simulink model "Openloop_voltage_control"  (R2020b)
settings: Solver=FixedStepDiscrete  StartTime=0.0  StopTime=Inf  RelTol=1e-3  EnableMultiTasking=on
values from neighbouring files (symbols this model uses):
  D_IGBT_CCM = (V_IGBT_out+V_diode_forward_drop-V_in)/(V_IGBT_out+V_diode_forward_drop)    (= 0.850746268657)    [Openloop_voltage_control_parameters.m]
  D_MOSFET_CCM = (V_MOSFET_out+V_diode_forward_drop-V_in)/(V_MOSFET_out+V_diode_forward_drop)    (= 0.70297029703)    [Openloop_voltage_control_parameters.m]
  Ki_IGBT = 0    [Openloop_voltage_control_parameters.m]
  Ki_MOSFET = 0    [Openloop_voltage_control_parameters.m]
  Kp_IGBT = 0    [Openloop_voltage_control_parameters.m]
  Kp_MOSFET = 0    [Openloop_voltage_control_parameters.m]
  Timer_period_IGBT = round(60e6/f_sw_IGBT)    [Openloop_voltage_control_parameters.m]
  Timer_period_MOSFET = round(60e6/f_sw_MOSFET)    [Openloop_voltage_control_parameters.m]
undefined symbols (not defined in the file or in its folder): GPTRIP1SEL, GPTRIP2SEL, TZ1, TZ2
undefined symbols (not defined in the file): C2000, Clear, Disable, ePWM2, ePWMxA, Immediate, Positive, Set, Up
libraries: c2802xlib x9, pid_lib x2, dspsigops x2, c280xlib x1
(part 1 of 2)
settings Model: ExtModeTrigDuration=8  Creator=Mladen  LastModifiedBy=hites
settings SolverCC: AutoInsertRateTranBlk=on
settings DataIOCC: ReturnWorkspaceOutputs=off
settings OptimizationCC: DefaultUnderspecifiedDataType=single  EnhancedBackFolding=on  PassReuseOutputArgsAs=Individual arguments  MaxStackSize=512  OptimizeBlockOrder=speed  DifferentSizesBufferReuse=on  OptimizationCustomize=off  EfficientTunableParamExpr=on
settings DebuggingCC: ParameterTunabilityLossMsg=error  ArithmeticOperatorsInVariantConditions=warning
settings HardwareCC: ProdBitPerChar=16  ProdBitPerInt=16  ProdBitPerPointer=32  ProdBitPerSizeT=32  ProdBitPerPtrDiffT=32  ProdLargestAtomicInteger=Integer  ProdLargestAtomicFloat=None  ProdWordSize=16  ProdLongLongMode=on  ProdHWDeviceType=Texas Instruments->C2000
settings SFSimCC: MATLABDynamicMemAlloc=off  CustomCodeUndefinedFunction=UseInterfaceOnly
settings RTWCC: Description=Embedded Coder  SystemTargetFile=ert.tlc  HardwareBoard=TI Piccolo F28027/F28027F LaunchPad  TemplateMakefile=ert_default_tmf  GenerateReport=on  Toolchain=Texas Instruments Code Composer Studio (C2000)  IncludeHyperlinkInReport=on  LaunchReport=on  GenerateTraceInfo=on  GenerateTraceReport=on  GenerateTraceReportSl=on  GenerateTraceReportSf=on  GenerateTraceReportEml=on
settings CodeAppCC: ForceParamTrailComments=on  IgnoreCustomStorageClasses=off  OperatorAnnotations=on  SimulinkDataObjDesc=on  SFDataObjDesc=on  InsertBlockDesc=on
settings ERTTargetCC: CodeReplacementLibrary=TI C28x

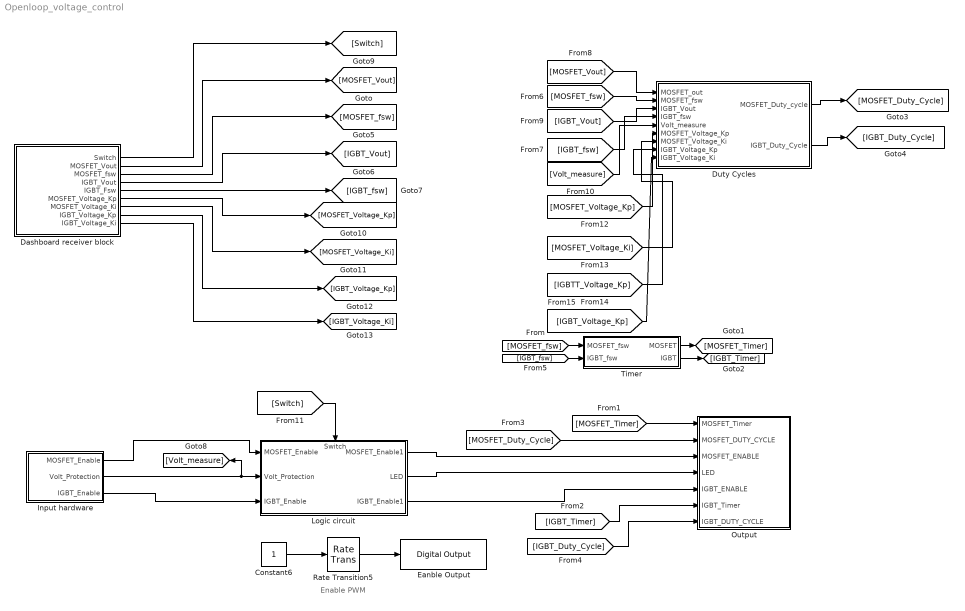
== system Openloop_voltage_control ==
  note: Enable PWM
  Constant6 : Constant  OutDataTypeStr=boolean  SampleTime=0.01
  Dashboard receiver block : Subsystem
  Duty Cycles : Subsystem
  Eanble Output : c2802xlib/Digital Output  GPIO_Number=GPIO0~GPIO7  GPIO_Bit0=off  GPIO_BIT0_Toggle=off  GPIO_Bit1=off  GPIO_BIT1_Toggle=off  GPIO_Bit2=off  GPIO_BIT2_Toggle=off  GPIO_Bit3=off  GPIO_BIT3_Toggle=off  GPIO_Bit4=on  GPIO_BIT4_Toggle=off  GPIO_Bit5=off  GPIO_BIT5_Toggle=off  GPIO_Bit6=off  GPIO_BIT6_Toggle=off  GPIO_Bit7=off  GPIO_BIT7_Toggle=off
      settings: SourceProductBaseCode=TIC2000
  Input hardware : Subsystem
  Logic circuit : Subsystem
      settings: PortSchema="{\"entries\":[{\"content\":{\"sides\":[{\"content\":{\"connectorIds\":[\"In1\",\"In2\",\"In3\"]},\"type\":\"ConnectorPlacement.EquallySpacedRectSide\",\"uuid\":\"9edef9f6-4e06-49ff-9487-f0c876c6db56\"},{\"content\":{\"connectorIds\":[\"Out1\",\"Out2\",\"Out3\"],\"side\":\"RIGHT\"},\"type\":\"ConnectorPlacement.EquallySpacedRectSide\",\"uuid\":\"38654259-1306-4cb6-b452-8646906e5123\"},{\"content\":{\"connectorIds\":[\"In4\"],\"side\":\"TOP\"},\"type\":\"ConnectorPlacement.EquallySpacedRectSide\",\"uuid\":\"81b5187c-2f62-4987-b311-955428575483\"},{\"content\":{\"connectorIds\":[],\"side\":\"HIDDEN\"},\"type\":\"ConnectorPlacement.EquallySpacedRectSide\",\"uuid\":\"52992d09-5af1-4048-a992-404c39f4bc87\"}]},\"type\":\"ConnectorPlacement.EquallySpacedConnector\",\"uuid\":\"3860a4b4-3099-482c-9336-e0768bc23cc0\"}],\"packageUris\":[\"http://schema.mathworks.com/mf0/Connector/R2020b\"],\"version\":\"1.0\"}"
  Output : Subsystem
  Rate Transition5 : RateTransition  Deterministic=off
  Timer : Subsystem
  wires:
  Constant6/1 -> Rate Transition5/1
  Rate Transition5/1 -> Eanble Output/1
  Duty Cycles/1(MOSFET_Duty_cycle) -> [MOSFET_Duty_Cycle]
  Duty Cycles/2(IGBT_Duty_Cycle) -> [IGBT_Duty_Cycle]
  Timer/1(MOSFET) -> [MOSFET_Timer]
  Timer/2(IGBT) -> [IGBT_Timer]
  Dashboard receiver block/2(MOSFET_Vout) -> [MOSFET_Vout]
  Dashboard receiver block/3(MOSFET_fsw) -> [MOSFET_fsw]
  Dashboard receiver block/4(IGBT_Vout) -> [IGBT_Vout]
  Dashboard receiver block/5(IGBT_Fsw) -> [IGBT_fsw]
  [MOSFET_fsw] -> Timer/1(MOSFET_fsw)
  [IGBT_fsw] -> Timer/2(IGBT_fsw)
  [MOSFET_Vout] -> Duty Cycles/1(MOSFET_out)
  [MOSFET_fsw] -> Duty Cycles/2(MOSFET_fsw)
  [IGBT_Vout] -> Duty Cycles/3(IGBT_Vout)
  [IGBT_fsw] -> Duty Cycles/4(IGBT_fsw)
  [Volt_measure] -> Duty Cycles/5(Volt_measure)
  Input hardware/2(Volt_Protection) -> [Volt_measure], Logic circuit/2(Volt_Protection)
  Input hardware/1(MOSFET_Enable) -> Logic circuit/1(MOSFET_Enable)
  Input hardware/3(IGBT_Enable) -> Logic circuit/3(IGBT_Enable)
  [MOSFET_Timer] -> Output/1(MOSFET_Timer)
  [MOSFET_Duty_Cycle] -> Output/2(MOSFET_DUTY_CYCLE)
  Logic circuit/1(MOSFET_Enable1) -> Output/3(MOSFET_ENABLE)
  Logic circuit/2(LED) -> Output/4(LED)
  Logic circuit/3(IGBT_Enable1) -> Output/5(IGBT_ENABLE)
  [IGBT_Timer] -> Output/6(IGBT_Timer)
  [IGBT_Duty_Cycle] -> Output/7(IGBT_DUTY_CYCLE)
  Dashboard receiver block/1(Switch) -> [Switch]
  Dashboard receiver block/6(MOSFET_Voltage_Kp) -> [MOSFET_Voltage_Kp]
  Dashboard receiver block/7(MOSFET_Voltage_Ki) -> [MOSFET_Voltage_Ki]
  Dashboard receiver block/8(IGBT_Voltage_Kp) -> [IGBT_Voltage_Kp]
  Dashboard receiver block/9(IGBT_Voltage_Ki) -> [IGBT_Voltage_Ki]
  [Switch] -> Logic circuit/4(Switch)
  [MOSFET_Voltage_Ki] -> Duty Cycles/7(MOSFET_Voltage_Ki)
  [MOSFET_Voltage_Kp] -> Duty Cycles/6(MOSFET_Voltage_Kp)
  [IGBTT_Voltage_Kp] -> Duty Cycles/8(IGBT_Voltage_Kp)
  [IGBT_Voltage_Kp] -> Duty Cycles/9(IGBT_Voltage_Ki)

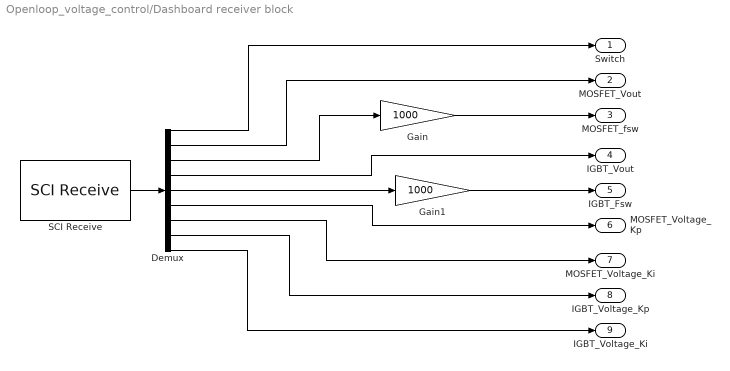
== system Openloop_voltage_control/Dashboard receiver block ==
  Demux : Demux  Outputs=9
  Gain : Gain  Gain=1000
  Gain1 : Gain  Gain=1000
  SCI Receive : c280xlib/SCI Receive  sciModule=A  dataHead='S'  dataTail='E'  dataType=uint16  dataDim=9  initValue=0  errOption=Output the last received value  errValue=0  sampleTime=-1  outputStatus=off  postInterrupt=off  numFifo=1
      settings: SourceProductName=Embedded Coder Support Package for Texas Instruments C2000 Processors
  Switch : Outport
  MOSFET_Vout : Outport  Port=2
  MOSFET_fsw : Outport  Port=3
  IGBT_Vout : Outport  Port=4
  IGBT_Fsw : Outport  Port=5
  MOSFET_Voltage_Kp : Outport  Port=6
  MOSFET_Voltage_Ki : Outport  Port=7
  IGBT_Voltage_Kp : Outport  Port=8
  IGBT_Voltage_Ki : Outport  Port=9
  wires:
  SCI Receive/1 -> Demux/1
  Gain/1 -> MOSFET_fsw/1
  Gain1/1 -> IGBT_Fsw/1
  Demux/5 -> Gain1/1
  Demux/4 -> IGBT_Vout/1
  Demux/3 -> Gain/1
  Demux/2 -> MOSFET_Vout/1
  Demux/1 -> Switch/1
  Demux/7 -> MOSFET_Voltage_Ki/1
  Demux/8 -> IGBT_Voltage_Kp/1
  Demux/9 -> IGBT_Voltage_Ki/1
  Demux/6 -> MOSFET_Voltage_Kp/1

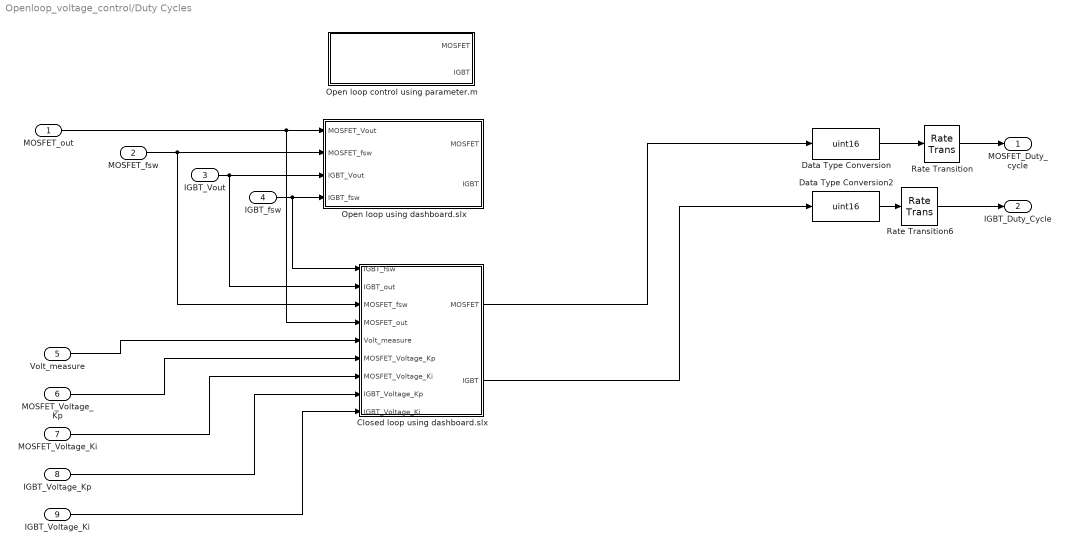
== system Openloop_voltage_control/Duty Cycles ==
  MOSFET_out : Inport
  MOSFET_fsw : Inport  Port=2
  IGBT_Vout : Inport  Port=3
  IGBT_fsw : Inport  Port=4
  Volt_measure : Inport  Port=5
  MOSFET_Voltage_Kp : Inport  Port=6
  MOSFET_Voltage_Ki : Inport  Port=7
  IGBT_Voltage_Kp : Inport  Port=8
  IGBT_Voltage_Ki : Inport  Port=9
  Closed loop using dashboard.slx : Subsystem
  Data Type Conversion : DataTypeConversion  OutDataTypeStr=uint16
  Data Type Conversion2 : DataTypeConversion  OutDataTypeStr=uint16
  Open loop control using parameter.m : Subsystem
  Open loop using dashboard.slx : Subsystem
  Rate Transition : RateTransition
  Rate Transition6 : RateTransition
  MOSFET_Duty_cycle : Outport
  IGBT_Duty_Cycle : Outport  Port=2
  wires:
  Data Type Conversion/1 -> Rate Transition/1
  Rate Transition/1 -> MOSFET_Duty_cycle/1
  Data Type Conversion2/1 -> Rate Transition6/1
  Rate Transition6/1 -> IGBT_Duty_Cycle/1
  MOSFET_out/1 -> Closed loop using dashboard.slx/4(MOSFET_out), Open loop using dashboard.slx/1(MOSFET_Vout)
  MOSFET_fsw/1 -> Closed loop using dashboard.slx/3(MOSFET_fsw), Open loop using dashboard.slx/2(MOSFET_fsw)
  IGBT_Vout/1 -> Closed loop using dashboard.slx/2(IGBT_out), Open loop using dashboard.slx/3(IGBT_Vout)
  IGBT_fsw/1 -> Closed loop using dashboard.slx/1(IGBT_fsw), Open loop using dashboard.slx/4(IGBT_fsw)
  Volt_measure/1 -> Closed loop using dashboard.slx/5(Volt_measure)
  MOSFET_Voltage_Kp/1 -> Closed loop using dashboard.slx/6(MOSFET_Voltage_Kp)
  MOSFET_Voltage_Ki/1 -> Closed loop using dashboard.slx/7(MOSFET_Voltage_Ki)
  IGBT_Voltage_Kp/1 -> Closed loop using dashboard.slx/8(IGBT_Voltage_Kp)
  IGBT_Voltage_Ki/1 -> Closed loop using dashboard.slx/9(IGBT_Voltage_Ki)
  Closed loop using dashboard.slx/1(MOSFET) -> Data Type Conversion/1
  Closed loop using dashboard.slx/2(IGBT) -> Data Type Conversion2/1

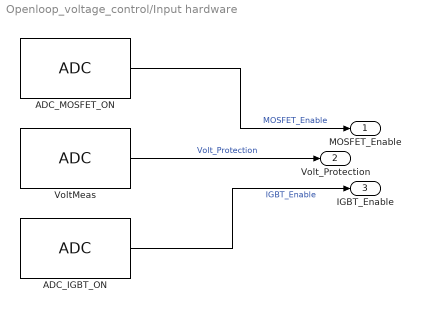
== system Openloop_voltage_control/Input hardware ==
  ADC_IGBT_ON : c2802xlib/ADC  blkParamProc=C2000  ADCModule=1  samplingMode=Single sample mode  ADCResolution=12-bit (Single-ended input)  useSOC1=SOC2  useSOC2=SOC0_SOC1  SOCAcquisitionWindow=7  SOCTriggerSource=Software  SOCInterruptTrigger=No ADCINT  Ts=0.001  dType=uint16  postInterrupt=off  interruptSel=ADCINT1  ADCINTContinuous=off  endma=off  chdma=1  conv1=ADCINA3  conv2=ADCINA7 and ADCINB7  conv1_Type4=ADCIN0  conv2_Type4=ADCIN0 and ADCIN1
  ADC_MOSFET_ON : c2802xlib/ADC  blkParamProc=C2000  ADCModule=1  samplingMode=Single sample mode  ADCResolution=12-bit (Single-ended input)  useSOC1=SOC0  useSOC2=SOC0_SOC1  SOCAcquisitionWindow=7  SOCTriggerSource=Software  SOCInterruptTrigger=No ADCINT  Ts=0.001  dType=uint16  postInterrupt=off  interruptSel=ADCINT1  ADCINTContinuous=off  endma=off  chdma=1  conv1=ADCINA7  conv2=ADCINA7 and ADCINB7  conv1_Type4=ADCIN0  conv2_Type4=ADCIN0 and ADCIN1
  VoltMeas : c2802xlib/ADC  blkParamProc=C2000  ADCModule=1  samplingMode=Single sample mode  ADCResolution=12-bit (Single-ended input)  useSOC1=SOC8  useSOC2=SOC0_SOC1  SOCAcquisitionWindow=7  SOCTriggerSource=Software  SOCInterruptTrigger=No ADCINT  Ts=0.001  dType=uint16  postInterrupt=off  interruptSel=ADCINT1  ADCINTContinuous=off  endma=off  chdma=1  conv1=ADCINB1  conv2=ADCINA7 and ADCINB7  conv1_Type4=ADCIN0  conv2_Type4=ADCIN0 and ADCIN1
  MOSFET_Enable : Outport
  Volt_Protection : Outport  Port=2
  IGBT_Enable : Outport  Port=3
  wires:
  ADC_MOSFET_ON/1 -> MOSFET_Enable/1  "MOSFET_Enable"
  VoltMeas/1 -> Volt_Protection/1  "Volt_Protection"
  ADC_IGBT_ON/1 -> IGBT_Enable/1  "IGBT_Enable"

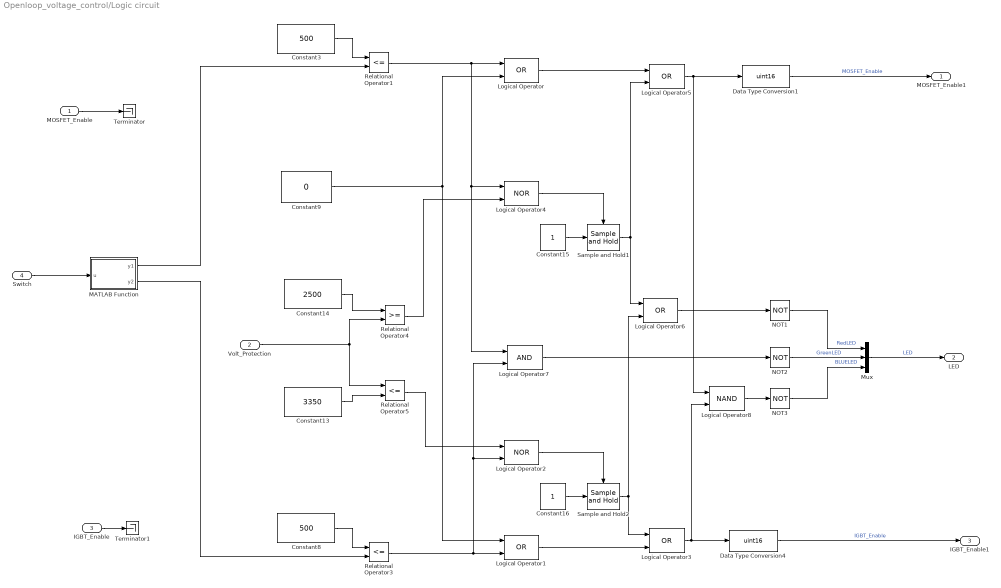
== system Openloop_voltage_control/Logic circuit ==
  MOSFET_Enable : Inport
  Volt_Protection : Inport  Port=2
  IGBT_Enable : Inport  Port=3
  Switch : Inport  Port=4
  Constant13 : Constant  Value=3350  OutDataTypeStr=uint16  SampleTime=-1
  Constant14 : Constant  Value=2500  OutDataTypeStr=uint16  SampleTime=-1
  Constant15 : Constant  OutDataTypeStr=boolean  SampleTime=-1
  Constant16 : Constant  OutDataTypeStr=boolean  SampleTime=-1
  Constant3 : Constant  Value=500  OutDataTypeStr=uint16  SampleTime=-1
  Constant8 : Constant  Value=500  OutDataTypeStr=uint16  SampleTime=-1
  Constant9 : Constant  Value=0  OutDataTypeStr=boolean  SampleTime=-1
  Data Type Conversion1 : DataTypeConversion  OutDataTypeStr=uint16
  Data Type Conversion4 : DataTypeConversion  OutDataTypeStr=uint16
  Logical Operator{,1,3,5..6} (5 alike) : Logic  Operator=OR  IconShape=distinctive  AllPortsSameDT=off  OutDataTypeStr=boolean
  Logical Operator2 : Logic  Operator=NOR  IconShape=distinctive  AllPortsSameDT=off  OutDataTypeStr=boolean
  Logical Operator4 : Logic  Operator=NOR  IconShape=distinctive  AllPortsSameDT=off  OutDataTypeStr=boolean
  Logical Operator7 : Logic  IconShape=distinctive  AllPortsSameDT=off  OutDataTypeStr=boolean
  Logical Operator8 : Logic  Operator=NAND  IconShape=distinctive  AllPortsSameDT=off  OutDataTypeStr=boolean
  MATLAB Function : MATLAB Function  TreatAsAtomicUnit=on
  Mux : Mux  Inputs=3
  NOT1 : Logic  Operator=NOT  IconShape=distinctive  AllPortsSameDT=off  OutDataTypeStr=boolean
  NOT2 : Logic  Operator=NOT  IconShape=distinctive  AllPortsSameDT=off  OutDataTypeStr=boolean
  NOT3 : Logic  Operator=NOT  IconShape=distinctive  AllPortsSameDT=off  OutDataTypeStr=boolean
  Relational Operator1 : RelationalOperator  Operator=<=  OutDataTypeStr=boolean  RndMeth=Simplest
  Relational Operator3 : RelationalOperator  Operator=<=  OutDataTypeStr=boolean  RndMeth=Simplest
  Relational Operator4 : RelationalOperator  OutDataTypeStr=boolean  RndMeth=Simplest
  Relational Operator5 : RelationalOperator  Operator=<=  OutDataTypeStr=boolean  RndMeth=Simplest
  Sample and Hold1 : dspsigops/Sample and Hold  trig=Rising edge  initCond=0  latchinput=off
  Sample and Hold2 : dspsigops/Sample and Hold  trig=Rising edge  initCond=0  latchinput=off
  Terminator : Terminator
  Terminator1 : Terminator
  MOSFET_Enable1 : Outport
  LED : Outport  Port=2
  IGBT_Enable1 : Outport  Port=3
  wires:
  Relational Operator1/1 -> Logical Operator7/1, Logical Operator4/1, Logical Operator/1
  Volt_Protection/1 -> Relational Operator4/2, Relational Operator5/1
  Logical Operator3/1 -> Data Type Conversion4/1, Logical Operator8/2
  Constant14/1 -> Relational Operator4/1
  Constant9/1 -> Logical Operator1/1, Logical Operator/2
  Logical Operator2/1 -> Sample and Hold2/Trigger
  Sample and Hold1/1 -> Logical Operator6/1, Logical Operator5/2
  Logical Operator5/1 -> Logical Operator8/1, Data Type Conversion1/1
  Constant15/1 -> Sample and Hold1/1
  Constant8/1 -> Relational Operator3/1
  Logical Operator8/1 -> NOT3/1
  Relational Operator3/1 -> Logical Operator7/2, Logical Operator2/2, Logical Operator1/2
  Data Type Conversion4/1 -> IGBT_Enable1/1  "IGBT_Enable"
  Logical Operator1/1 -> Logical Operator3/2
  Relational Operator4/1 -> Logical Operator4/2
  Logical Operator/1 -> Logical Operator5/1
  Relational Operator5/1 -> Logical Operator2/1
  Logical Operator4/1 -> Sample and Hold1/Trigger
  Sample and Hold2/1 -> Logical Operator3/1, Logical Operator6/2
  Constant3/1 -> Relational Operator1/1
  Constant16/1 -> Sample and Hold2/1
  Logical Operator7/1 -> NOT2/1
  Logical Operator6/1 -> NOT1/1
  Data Type Conversion1/1 -> MOSFET_Enable1/1  "MOSFET_Enable"
  NOT1/1 -> Mux/1  "RedLED"
  NOT2/1 -> Mux/2  "GreenLED"
  NOT3/1 -> Mux/3  "BLUELED"
  Mux/1 -> LED/1  "LED"
  Constant13/1 -> Relational Operator5/2
  Switch/1 -> MATLAB Function/1(u)
  MOSFET_Enable/1 -> Terminator/1
  IGBT_Enable/1 -> Terminator1/1
  MATLAB Function/1(y1) -> Relational Operator1/2
  MATLAB Function/2(y2) -> Relational Operator3/2

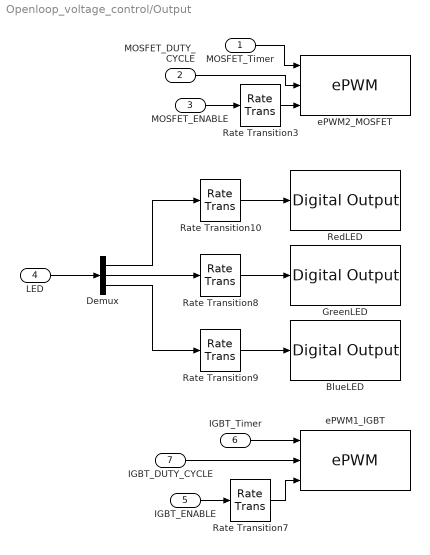
== system Openloop_voltage_control/Output ==
  MOSFET_Timer : Inport
  MOSFET_DUTY_CYCLE : Inport  Port=2
  MOSFET_ENABLE : Inport  Port=3
  LED : Inport  Port=4
  IGBT_ENABLE : Inport  Port=5
  IGBT_Timer : Inport  Port=6
  IGBT_DUTY_CYCLE : Inport  Port=7
  BlueLED : c2802xlib/Digital Output  GPIO_Number=GPIO8~GPIO15  GPIO_Bit0=off  GPIO_BIT0_Toggle=off  GPIO_Bit1=off  GPIO_BIT1_Toggle=off  GPIO_Bit2=off  GPIO_BIT2_Toggle=off  GPIO_Bit3=off  GPIO_BIT3_Toggle=off  GPIO_Bit4=on  GPIO_BIT4_Toggle=off  GPIO_Bit5=off  GPIO_BIT5_Toggle=off  GPIO_Bit6=off  GPIO_BIT6_Toggle=off  GPIO_Bit7=off  GPIO_BIT7_Toggle=off
      settings: SourceProductBaseCode=TIC2000
  Demux : Demux  Outputs=3
  GreenLED : c2802xlib/Digital Output  GPIO_Number=GPIO16~GPIO23  GPIO_Bit0=off  GPIO_BIT0_Toggle=off  GPIO_Bit1=off  GPIO_BIT1_Toggle=off  GPIO_Bit2=off  GPIO_BIT2_Toggle=off  GPIO_Bit3=on  GPIO_BIT3_Toggle=off  GPIO_Bit4=off  GPIO_BIT4_Toggle=off  GPIO_Bit5=off  GPIO_BIT5_Toggle=off  GPIO_Bit6=off  GPIO_BIT6_Toggle=off  GPIO_Bit7=off  GPIO_BIT7_Toggle=off
      settings: SourceProductBaseCode=TIC2000
  Rate Transition10 : RateTransition  Deterministic=off
  Rate Transition3 : RateTransition
  Rate Transition7 : RateTransition
  Rate Transition8 : RateTransition  Deterministic=off  InitialCondition=1
  Rate Transition9 : RateTransition  Deterministic=off
  RedLED : c2802xlib/Digital Output  GPIO_Number=GPIO32~GPIO34  GPIO_Bit0=off  GPIO_BIT0_Toggle=off  GPIO_Bit1=off  GPIO_BIT1_Toggle=off  GPIO_Bit2=on  GPIO_BIT2_Toggle=off  GPIO_Bit3=off  GPIO_BIT3_Toggle=off  GPIO_Bit4=off  GPIO_BIT4_Toggle=off  GPIO_Bit5=off  GPIO_BIT5_Toggle=off  GPIO_Bit6=off  GPIO_BIT6_Toggle=off  GPIO_Bit7=off  GPIO_BIT7_Toggle=off
      settings: SourceProductBaseCode=TIC2000
  ePWM1_IGBT : c2802xlib/ePWM  PwmType=C2000  useModule=ePWM1  ePWMxLINKTBPRD=Not Linked  periodUnits=Clock cycles  timerSource=Input port  timerPeriod_clk=Timer_period_IGBT*2  timerPeriod_sec=0.0001  tbshadow=Counter equals to zero  countingMode=Up  phaseActiveEnable=Disable  phaseDirection=Count down after sync  phaseActive=0  synchronizationEnable=off  dcaevt1Sync=off  dcbevt1Sync=off  synchronizationOption=Disable  perSynchronizationOption=Counter equals to period (CTR=PRD)  clockPrescale=1  HSclockPrescale=1  enswap=off  ePWMxAStatus=on  ePWMxAactionLogic1=Set  ePWMxAactionLogic2=Set  ePWMxAactionLogic3=Clear  ePWMxAactionLogic4=Set  ePWMxAactionLogic5=Do nothing  ePWMxAactionLogic6=Do nothing  ePWMxACSFenable=on  ePWMxACSFvalue=Forcing disable  ePWMxASFreload=Immediate  ePWMxBStatus=off  ePWMxBactionLogic1=Set  ePWMxBactionLogic2=Clear  ePWMxBactionLogic3=Do nothing  ePWMxBactionLogic4=Do nothing  ePWMxBactionLogic5=Clear  ePWMxBactionLogic6=Set  ePWMxBCSFenable=off  ePWMxBCSFvalue=Forcing disable  ePWMxBSFreload=Immediate  ePWNxBOutWay=off  ePWMxLINKCMPA=Not Linked  CMPAUnits=Clock cycles  CMPASource=Input port  CMPAValue_per=50  CMPAValue_clk=2000  enCMPAshadow=Counter equals to zero (CTR=Zero)  ePWMxLINKCMPB=Not Linked  CMPBUnits=Clock cycles  CMPBSource=Specify via dialog  CMPBValue_per=50  CMPBValue_clk=32000  enCMPBshadow=Counter equals to zero (CTR=Zero)  ePWMxLINKCMPC=Not Linked  CMPCUnits=Clock cycles  CMPCSource=Specify via dialog  CMPCValue_per=50  CMPCValue_clk=32000  enCMPCshadow=Counter equals to zero (CTR=Zero)  ePWMxLINKCMPD=Not Linked  CMPDUnits=Clock cycles  CMPDSource=Specify via dialog  CMPDValue_per=50  CMPDValue_clk=32000  enCMPDshadow=Counter equals to zero (CTR=Zero)  enableDBePWMxA=off  enableDBePWMxB=off  enhalfcycle=off  DBpolarity=Active high (AH)  DBedgeDelay=Positive  DBSource_ePWMxA=ePWMxA  DBSource_ePWMxB=ePWMxA  DBPeriodUnits=Clock cycles  DBperiodSource=Specify via dialog  REDperiod=0  FEDperiod=0  REDperiod_sec=0  FEDperiod_sec=0  LoadModeDBRED=Immediate without using shadow  LoadModeDBFED=Immediate without using shadow  adcstartModuleA=off  adcrequestEventA=First event  adcstartEventA=Digital Compare Module A Event 1 start of conversion (DCAEVT1.soc)  adcstartEventA_type2=Digital Compare Module A Event 1 start of conversion (DCAEVT1.soc)  adcstartModuleB=off  adcrequestEventB=First event  adcstartEventB=Counter equals to zero (CTR=Zero)  adcstartEventB_type2=Counter equals to zero (CTR=Zero)  intEn=off  intPrd=First event  intSel=Counter equals to zero (CTR=Zero)  intSel_type2=Counter equals to zero (CTR=Zero)  hrpe=off  enHRPWM=off  HRPWM_LoadMode=Counter equals to period (CTR=PRD)  HRPWM_CTLMode=Duty or Period control mode  HRPWM_EDGMode=Both edge  hrpeb=off  enHRPWMB=off  HRPWM_LoadModeB=Counter equals to zero (CTR=ZERO)  HRPWM_CTLModeB=Duty or Period control mode  HRPWM_EDGModeB=Both edge  enHRDBRED=off  enHRDBFED=off  enSFO=on  enautoconv=on  chopperEnable=off  chopperFrequency=1  chopperFirstwidth=1  chopperDuty=12.5%  tripZonesource=Specify via dialog  tzselOSHT1=off  tzselOSHT2=off  tzselOSHT3=off  tzselOSHDCAEV1=off  tzselOSHDCBEV1=off  tzselCBC1=off  tzselCBC2=off  tzselCBC3=off  tzselCBCDCAEV2=off  tzselCBCDCBEV2=off  tzselOSHT4=off  tzselOSHT5=off  tzselOSHT6=off  tzselCBC4=off  tzselCBC5=off  tzselCBC6=off  enTzOstIntr=off  enTzCbcIntr=off  enTzDCAEVT1Intr=off  enTzDCAEVT2Intr=off  enTzDCBEVT1Intr=off  enTzDCBEVT2Intr=off  ePWMxAforced=No action  ePWMxBforced=No action  DCAEVT1forced=No action  DCBEVT1forced=No action  DCAEVT2forced=No action  DCBEVT2forced=No action  dcah=Trip Zone 1 input (TZ1)  dcal=Trip Zone 2 input (TZ2)  dcbh=Trip Zone 1 input (TZ1)  dcbl=Trip Zone 2 input (TZ2)  dcah_type2=GPTRIP1SEL/(TZ1)  dcal_type2=GPTRIP2SEL/(TZ2)  dcbh_type2=GPTRIP1SEL/(TZ1)  dcbl_type2=GPTRIP2SEL/(TZ2)  gendcaevt1=Event disabled  gendcaevt2=Event disabled  gendcbevt1=Event disabled  gendcbevt2=Event disabled  dcaevt1src=DCAEVT1 with sync  dcaevt2src=DCAEVT2 with sync  dcbevt1src=DCBEVT1 with sync  dcbevt2src=DCBEVT2 with sync  pulsesel=Counter equals to zero (CTR=Zero)  blankinv=off  blankoffset=0  blankwidth=0  evsrcsel=Filtered version of DCAEVT1 (DCAEVT1FILT)  encape=off
  ePWM2_MOSFET : c2802xlib/ePWM  PwmType=C2000  useModule=ePWM2  ePWMxLINKTBPRD=Not Linked  periodUnits=Clock cycles  timerSource=Input port  timerPeriod_clk=timerPeriod_clk  timerPeriod_sec=timerPeriod_sec  tbshadow=Counter equals to zero  countingMode=Up  phaseActiveEnable=Disable  phaseDirection=Count down after sync  phaseActive=phaseActive  synchronizationEnable=off  dcaevt1Sync=off  dcbevt1Sync=off  synchronizationOption=Disable  perSynchronizationOption=Counter equals to period (CTR=PRD)  clockPrescale=1  HSclockPrescale=1  enswap=off  ePWMxAStatus=on  ePWMxAactionLogic1=Set  ePWMxAactionLogic2=Set  ePWMxAactionLogic3=Clear  ePWMxAactionLogic4=Set  ePWMxAactionLogic5=Do nothing  ePWMxAactionLogic6=Do nothing  ePWMxACSFenable=on  ePWMxACSFvalue=Forcing disable  ePWMxASFreload=Immediate  ePWMxBStatus=off  ePWMxBactionLogic1=Set  ePWMxBactionLogic2=Clear  ePWMxBactionLogic3=Do nothing  ePWMxBactionLogic4=Do nothing  ePWMxBactionLogic5=Clear  ePWMxBactionLogic6=Set  ePWMxBCSFenable=off  ePWMxBCSFvalue=Forcing disable  ePWMxBSFreload=Immediate  ePWNxBOutWay=off  ePWMxLINKCMPA=Not Linked  CMPAUnits=Clock cycles  CMPASource=Input port  CMPAValue_per=CMPAValue_per  CMPAValue_clk=CMPAValue_clk  enCMPAshadow=Counter equals to zero (CTR=Zero)  ePWMxLINKCMPB=Not Linked  CMPBUnits=Clock cycles  CMPBSource=Specify via dialog  CMPBValue_per=CMPBValue_per  CMPBValue_clk=CMPBValue_clk  enCMPBshadow=Counter equals to zero (CTR=Zero)  ePWMxLINKCMPC=Not Linked  CMPCUnits=Clock cycles  CMPCSource=Specify via dialog  CMPCValue_per=CMPCValue_per  CMPCValue_clk=CMPCValue_clk  enCMPCshadow=Counter equals to zero (CTR=Zero)  ePWMxLINKCMPD=Not Linked  CMPDUnits=Clock cycles  CMPDSource=Specify via dialog  CMPDValue_per=CMPDValue_per  CMPDValue_clk=CMPDValue_clk  enCMPDshadow=Counter equals to zero (CTR=Zero)  enableDBePWMxA=off  enableDBePWMxB=off  enhalfcycle=off  DBpolarity=Active high (AH)  DBedgeDelay=Positive  DBSource_ePWMxA=ePWMxA  DBSource_ePWMxB=ePWMxA  DBPeriodUnits=Clock cycles  DBperiodSource=Specify via dialog  REDperiod=REDperiod  FEDperiod=FEDperiod  REDperiod_sec=REDperiod_sec  FEDperiod_sec=FEDperiod_sec  LoadModeDBRED=Immediate without using shadow  LoadModeDBFED=Immediate without using shadow  adcstartModuleA=off  adcrequestEventA=First event  adcstartEventA=Digital Compare Module A Event 1 start of conversion (DCAEVT1.soc)  adcstartEventA_type2=Digital Compare Module A Event 1 start of conversion (DCAEVT1.soc)  adcstartModuleB=off  adcrequestEventB=First event  adcstartEventB=Counter equals to zero (CTR=Zero)  adcstartEventB_type2=Counter equals to zero (CTR=Zero)  intEn=off  intPrd=First event  intSel=Counter equals to zero (CTR=Zero)  intSel_type2=Counter equals to zero (CTR=Zero)  hrpe=off  enHRPWM=off  HRPWM_LoadMode=Counter equals to period (CTR=PRD)  HRPWM_CTLMode=Duty or Period control mode  HRPWM_EDGMode=Both edge  hrpeb=off  enHRPWMB=off  HRPWM_LoadModeB=Counter equals to zero (CTR=ZERO)  HRPWM_CTLModeB=Duty or Period control mode  HRPWM_EDGModeB=Both edge  enHRDBRED=off  enHRDBFED=off  enSFO=on  enautoconv=on  chopperEnable=off  chopperFrequency=1  chopperFirstwidth=1  chopperDuty=12.5%  tripZonesource=Specify via dialog  tzselOSHT1=off  tzselOSHT2=off  tzselOSHT3=off  tzselOSHDCAEV1=off  tzselOSHDCBEV1=off  tzselCBC1=off  tzselCBC2=off  tzselCBC3=off  tzselCBCDCAEV2=off  tzselCBCDCBEV2=off  tzselOSHT4=off  tzselOSHT5=off  tzselOSHT6=off  tzselCBC4=off  tzselCBC5=off  tzselCBC6=off  enTzOstIntr=off  enTzCbcIntr=off  enTzDCAEVT1Intr=off  enTzDCAEVT2Intr=off  enTzDCBEVT1Intr=off  enTzDCBEVT2Intr=off  ePWMxAforced=No action  ePWMxBforced=No action  DCAEVT1forced=No action  DCBEVT1forced=No action  DCAEVT2forced=No action  DCBEVT2forced=No action  dcah=Trip Zone 1 input (TZ1)  dcal=Trip Zone 2 input (TZ2)  dcbh=Trip Zone 1 input (TZ1)  dcbl=Trip Zone 2 input (TZ2)  dcah_type2=GPTRIP1SEL/(TZ1)  dcal_type2=GPTRIP2SEL/(TZ2)  dcbh_type2=GPTRIP1SEL/(TZ1)  dcbl_type2=GPTRIP2SEL/(TZ2)  gendcaevt1=Event disabled  gendcaevt2=Event disabled  gendcbevt1=Event disabled  gendcbevt2=Event disabled  dcaevt1src=DCAEVT1 with sync  dcaevt2src=DCAEVT2 with sync  dcbevt1src=DCBEVT1 with sync  dcbevt2src=DCBEVT2 with sync  pulsesel=Counter equals to zero (CTR=Zero)  blankinv=off  blankoffset=blankoffset  blankwidth=blankwidth  evsrcsel=Filtered version of DCAEVT1 (DCAEVT1FILT)  encape=off  mask(C2802x/03x/05x/06x/M3x/37x/07x/004x/38x ePWM){PwmType=C2000, useModule=ePWM2, ePWMxLINKTBPRD=Not Linked, periodUnits=Clock cycles, timerSource=Input port, timerPeriod_clk=Timer_period_MOSFET*2, timerPeriod_sec=0.0001, tbshadow=Counter equals to zero, countingMode=Up, phaseActiveEnable=Disable, phaseDirection=Count down after sync, phaseActive=0, synchronizationEnable=off, dcaevt1Sync=off, dcbevt1Sync=off, synchronizationOption=Disable, perSynchronizationOption=Counter equals to period (CTR=PRD), clockPrescale=1, HSclockPrescale=1, enswap=off, ePWMxAStatus=on, ePWMxAactionLogic1=Set, ePWMxAactionLogic2=Set, ePWMxAactionLogic3=Clear, ePWMxAactionLogic4=Set, ePWMxAactionLogic5=Do nothing, ePWMxAactionLogic6=Do nothing, ePWMxACSFenable=on, ePWMxACSFvalue=Forcing disable, ePWMxASFreload=Immediate, ePWMxBStatus=off, ePWMxBactionLogic1=Set, ePWMxBactionLogic2=Clear, ePWMxBactionLogic3=Do nothing, ePWMxBactionLogic4=Do nothing, ePWMxBactionLogic5=Clear, ePWMxBactionLogic6=Set, ePWMxBCSFenable=off, ePWMxBCSFvalue=Forcing disable, ePWMxBSFreload=Immediate, ePWNxBOutWay=off, ePWMxLINKCMPA=Not Linked, CMPAUnits=Clock cycles, CMPASource=Input port, CMPAValue_per=50, CMPAValue_clk=525, enCMPAshadow=Counter equals to zero (CTR=Zero), ePWMxLINKCMPB=Not Linked, CMPBUnits=Clock cycles, CMPBSource=Specify via dialog, CMPBValue_per=50, CMPBValue_clk=32000, enCMPBshadow=Counter equals to zero (CTR=Zero), ePWMxLINKCMPC=Not Linked, CMPCUnits=Clock cycles, CMPCSource=Specify via dialog, CMPCValue_per=50, CMPCValue_clk=32000, enCMPCshadow=Counter equals to zero (CTR=Zero), ePWMxLINKCMPD=Not Linked, CMPDUnits=Clock cycles, CMPDSource=Specify via dialog, CMPDValue_per=50, CMPDValue_clk=32000, enCMPDshadow=Counter equals to zero (CTR=Zero), enableDBePWMxA=off, enableDBePWMxB=off, enhalfcycle=off, DBpolarity=Active high (AH), DBedgeDelay=Positive, DBSource_ePWMxA=ePWMxA, DBSource_ePWMxB=ePWMxA, DBPeriodUnits=Clock cycles, DBperiodSource=Specify via dialog, REDperiod=0, FEDperiod=0, REDperiod_sec=0, FEDperiod_sec=0, LoadModeDBRED=Immediate without using shadow, LoadModeDBFED=Immediate without using shadow, adcstartModuleA=off, adcrequestEventA=First event, adcstartEventA=Digital Compare Module A Event 1 start of conversion (DCAEVT1.soc), adcstartEventA_type2=Digital Compare Module A Event 1 start of conversion (DCAEVT1.soc), adcstartModuleB=off, adcrequestEventB=First event, adcstartEventB=Counter equals to zero (CTR=Zero), adcstartEventB_type2=Counter equals to zero (CTR=Zero), intEn=off, intPrd=First event, intSel=Counter equals to zero (CTR=Zero), intSel_type2=Counter equals to zero (CTR=Zero), hrpe=off, enHRPWM=off, HRPWM_LoadMode=Counter equals to period (CTR=PRD), HRPWM_CTLMode=Duty or Period control mode, HRPWM_EDGMode=Both edge, hrpeb=off, enHRPWMB=off, HRPWM_LoadModeB=Counter equals to zero (CTR=ZERO), HRPWM_CTLModeB=Duty or Period control mode, HRPWM_EDGModeB=Both edge, enHRDBRED=off, enHRDBFED=off, enSFO=on, enautoconv=on, chopperEnable=off, chopperFrequency=1, chopperFirstwidth=1, chopperDuty=12.5%, tripZonesource=Specify via dialog, tzselOSHT1=off, tzselOSHT2=off, tzselOSHT3=off, tzselOSHDCAEV1=off, tzselOSHDCBEV1=off, tzselCBC1=off, tzselCBC2=off, tzselCBC3=off, tzselCBCDCAEV2=off, tzselCBCDCBEV2=off, tzselOSHT4=off, tzselOSHT5=off, tzselOSHT6=off, tzselCBC4=off, tzselCBC5=off, tzselCBC6=off, enTzOstIntr=off, enTzCbcIntr=off, enTzDCAEVT1Intr=off, enTzDCAEVT2Intr=off, enTzDCBEVT1Intr=off, enTzDCBEVT2Intr=off, ePWMxAforced=No action, ePWMxBforced=No action, DCAEVT1forced=No action, DCBEVT1forced=No action, DCAEVT2forced=No action, DCBEVT2forced=No action, dcah=Trip Zone 1 input (TZ1), dcal=Trip Zone 2 input (TZ2), dcbh=Trip Zone 1 input (TZ1), dcbl=Trip Zone 2 input (TZ2), dcah_type2=GPTRIP1SEL/(TZ1), dcal_type2=GPTRIP2SEL/(TZ2), dcbh_type2=GPTRIP1SEL/(TZ1), dcbl_type2=GPTRIP2SEL/(TZ2), gendcaevt1=Event disabled, gendcaevt2=Event disabled, gendcbevt1=Event disabled, gendcbevt2=Event disabled, dcaevt1src=DCAEVT1 with sync, dcaevt2src=DCAEVT2 with sync, dcbevt1src=DCBEVT1 with sync, dcbevt2src=DCBEVT2 with sync, pulsesel=Counter equals to zero (CTR=Zero), blankinv=off, blankoffset=0, blankwidth=0, evsrcsel=Filtered version of DCAEVT1 (DCAEVT1FILT), encape=off}
      mask prompts: PwmType "BlockParameterProcessor"; useModule "Module:"; ePWMxLINKTBPRD "ePWMLink TBPRD"; periodUnits "Timer period units:"; timerSource "Specify timer period via:"; timerPeriod_clk "Timer period:"; timerPeriod_sec "Timer period:"; tbshadow "Reload for time base period register (PRDLD):"; countingMode "Counting mode:"; phaseActiveEnable "Synchronization action:"; phaseDirection "Counting direction after phase synchronization:"; phaseActive "Phase offset value (TBPHS):"; synchronizationEnable "Specify software synchronization via input port (SWFSYNC)"; dcaevt1Sync "Enable digital compare A event1 synchronization (DCAEVT1)"; dcbevt1Sync "Enable digital compare B event1 synchronization (DCBEVT1)"; synchronizationOption "Synchronization output (SYNCO):"; perSynchronizationOption "Peripheral synchronization event (PWMSYNCSEL):"; clockPrescale "Time base clock (TBCLK) prescaler divider:"; HSclockPrescale "High speed time base clock (HSPCLKDIV) prescaler divider:"; enswap "Enable swap module A and B"; ePWMxAStatus "Enable ePWM2A"; ePWMxAactionLogic1 "Action when counter=ZERO:"; ePWMxAactionLogic2 "Action when counter=period (PRD):"; ePWMxAactionLogic3 "Action when counter=CMPA on up-count (CAU):"; ePWMxAactionLogic4 "Action when counter=CMPA on down-count (CAD):"; ePWMxAactionLogic5 "Action when counter=CMPB on up-count (CBU):"; ePWMxAactionLogic6 "Action when counter=CMPB on down-count (CBD):"; ePWMxACSFenable "Add continuous software force input port"; ePWMxACSFvalue "Continuous software force logic:"; ePWMxASFreload "Reload condition for software force:"; ePWMxBStatus "Enable ePWM2B"; ePWMxBactionLogic1 "Action when counter=ZERO:"; ePWMxBactionLogic2 "Action when counter=period (PRD):"; ePWMxBactionLogic3 "Action when counter=CMPA on up-count (CAU):"; ePWMxBactionLogic4 "Action when counter=CMPA on down-count (CAD):"; ePWMxBactionLogic5 "Action when counter=CMPB on up-count (CBU):"; ePWMxBactionLogic6 "Action when counter=CMPB on down-count (CBD):"; ePWMxBCSFenable "Add continuous software force input port"; ePWMxBCSFvalue "Continuous software force logic:"; ePWMxBSFreload "Reload condition for software force:"; ePWNxBOutWay "Inverted version of ePWMxA"; ePWMxLINKCMPA "ePWMLink CMPA"; CMPAUnits "CMPA units:"; CMPASource "Specify CMPA via:"; CMPAValue_per "CMPA initial value:"; CMPAValue_clk "CMPA initial value:"; enCMPAshadow "Reload for compare A Register (SHDWAMODE):"; ePWMxLINKCMPB "ePWMLink CMPB"; CMPBUnits "CMPB units:"; CMPBSource "Specify CMPB via:"; CMPBValue_per "CMPB value:"; CMPBValue_clk "CMPB value:"; enCMPBshadow "Reload for compare B Register (SHDWBMODE):"; ePWMxLINKCMPC "ePWMLink CMPC"; CMPCUnits "CMPC units:"; CMPCSource "Specify CMPC via:"; CMPCValue_per "CMPC value:"; CMPCValue_clk "CMPC value:"; enCMPCshadow "Reload for compare C Register (SHDWCMODE):"; ePWMxLINKCMPD "ePWMLink CMPD"; CMPDUnits "CMPD units:"; CMPDSource "Specify CMPD via:"; CMPDValue_per "CMPD value:"; CMPDValue_clk "CMPD value:"; enCMPDshadow "Reload for compare D Register (SHDWDMODE):"; enableDBePWMxA "Use deadband for ePWM2A"; enableDBePWMxB "Use deadband for ePWM2B"; enhalfcycle "Enable half-cycle clocking"; DBpolarity "Deadband polarity:"; DBedgeDelay "Deadband polarity:"; DBSource_ePWMxA "Signal source for raising edge (RED):"; DBSource_ePWMxB "Signal source for falling edge (FED):"; DBPeriodUnits "Deadband period units:"; DBperiodSource "Deadband period source:"; REDperiod "Deadband Rising edge (RED) period (0~1023):"; FEDperiod "Deadband Falling edge (FED) period (0~1023):"; REDperiod_sec "Deadband Rising edge (RED) period:"; FEDperiod_sec "Deadband Falling edge (FED) period:"; LoadModeDBRED "Reload for DBRED register (SHDWDBRED):"; LoadModeDBFED "Reload for DBFED register (SHDWDBFED):"; adcstartModuleA "Enable ADC start of conversion for module A"; adcrequestEventA "Number of event for start of conversion A (SOCA) to be generated:"; adcstartEventA "Start of conversion for module A event selection:"; adcstartEventA_type2 "Start of conversion for module A event selection:"; adcstartModuleB "Enable ADC start of conversion for module B"; adcrequestEventB "Number of event for start of conversion B (SOCB) to be generated:"; adcstartEventB "Start of conversion for module B event selection:"; adcstartEventB_type2 "Start of conversion for module B event selection:"; intEn "Enable ePWM interrupt"; intPrd "Number of event for interrupt to be generated:"; intSel "Interrupt counter match event condition:"; intSel_type2 "Interrupt counter match event condition:"; hrpe "Enable High Resolution Period on ePWMxA(HRPWM-period)"; enHRPWM "Enable HRPWM Duty on ePWMxA(HRPWM-duty)"; HRPWM_LoadMode "High resolution PWM (HRPWM) Load mode on ePWMxA:"; HRPWM_CTLMode "High resolution PWM (HRPWM) control mode on ePWMxA:"; HRPWM_EDGMode "High resolution PWM (HRPWM) edge control mode on ePWMxA:"; hrpeb "Enable High Resolution Period on ePWMxB (HRPWM-period)"; enHRPWMB "Enable HRPWM Duty on ePWMxB (HRPWM-duty)"; HRPWM_LoadModeB "High resolution PWM (HRPWM) Load mode on ePWMxB:"; HRPWM_CTLModeB "High resolution PWM (HRPWM) control mode on ePWMxB:"; HRPWM_EDGModeB "High resolution PWM (HRPWM) edge control mode on ePWMxB:"; enHRDBRED "Enable high resolution deadband rising edge (RED)"; enHRDBFED "Enable high resolution deadband falling edge (FED)"; enSFO "Use scale factor optimizer (SFO) software"; enautoconv "Enable auto convert"; chopperEnable "Chopper module enable"; chopperFrequency "Chopper frequency divider:"; chopperFirstwidth "Chopper clock cycles width of first pulse:"; chopperDuty "Chopper pulse duty cycle:"; tripZonesource "Trip zone source:"; tzselOSHT1 "Enable one-shot trip-zone1 (TZ1)"; tzselOSHT2 "Enable one-shot trip-zone2 (TZ2)"; tzselOSHT3 "Enable one-shot trip-zone3 (TZ3)"; tzselOSHDCAEV1 "Enable one-shot digital compare A event 1 (DCAEVT1)"; tzselOSHDCBEV1 "Enable one-shot digital compare B event 1 (DCBEVT1)"; tzselCBC1 "Enable cyclic trip-zone1 (TZ1)"; tzselCBC2 "Enable cyclic trip-zone2 (TZ2)"; tzselCBC3 "Enable cyclic trip-zone3 (TZ3)"; tzselCBCDCAEV2 "Enable cyclic digital compare A event 2 (DCAEVT2)"; tzselCBCDCBEV2 "Enable cyclic digital compare B event 2 (DCBEVT2)"; tzselOSHT4 "Enable one-shot trip-zone4 (TZ4)"; tzselOSHT5 "Enable one-shot trip-zone5 (TZ5)"; tzselOSHT6 "Enable one-shot trip-zone6 (TZ6)"; tzselCBC4 "Enable cyclic trip-zone4 (TZ4)"; tzselCBC5 "Enable cyclic trip-zone5 (TZ5)"; tzselCBC6 "Enable cyclic trip-zone6 (TZ6)"; enTzOstIntr "Enable trip-zone one-shot interrupt (OST)"; enTzCbcIntr "Enable trip-zone cycle-by-cycle interrupt (CBC)"; enTzDCAEVT1Intr "Digital comparator output A event 1 interrupt enable (DCAEVT1)"; enTzDCAEVT2Intr "Digital comparator output A event 2 interrupt enable (DCAEVT2)"; enTzDCBEVT1Intr "Digital comparator output B event 1 interrupt enable (DCBEVT1)"; enTzDCBEVT2Intr "Digital comparator output B event 2 interrupt enable (DCBEVT2)"; ePWMxAforced "ePWM2A forced (TZ) to:"; ePWMxBforced "ePWM2B forced (TZ) to:"; DCAEVT1forced "ePWM2A forced (DCAEVT1) to:"; DCBEVT1forced "ePWM2B forced (DCBEVT1) to:"; DCAEVT2forced "ePWM2A forced (DCAEVT2) to:"; DCBEVT2forced "ePWM2B forced (DCBEVT2) to:"; dcah "Source for digital compare A high signal (DCAH):"; dcal "Source for digital compare A low signal (DCAL):"; dcbh "Source for digital compare B high signal (DCBH):"; dcbl "Source for digital compare B low signal (DCBL):"; dcah_type2 "Source for digital compare A high signal (DCAH):"; dcal_type2 "Source for digital compare A low signal (DCAL):"; dcbh_type2 "Source for digital compare B high signal (DCBH):"; dcbl_type2 "Source for digital compare B low signal (DCBL):"; gendcaevt1 "Digital compare output A event 1 selection (DCAEVT1):"; gendcaevt2 "Digital compare output A event 2 selection (DCAEVT2):"; gendcbevt1 "Digital compare output B event 1 selection (DCBEVT1):"; gendcbevt2 "Digital compare cutput B event 2 selection (DCBEVT2):"; dcaevt1src "DCAEVT1 source select:"; dcaevt2src "DCAEVT2 source select:"; dcbevt1src "DCBEVT1 source select:"; dcbevt2src "DCBEVT2 source select:"; pulsesel "Pulse select:"; blankinv "Blanking window inverted"; blankoffset "Blanking window offset"; blankwidth "Blanking window width"; evsrcsel "Filter source select:"; encape "Enable counter capture"
      mask TypeOptions PwmType: PwmType
      mask TypeOptions useModule: useModule
      mask TypeOptions ePWMxLINKTBPRD: ePWMxLINKTBPRD
      mask TypeOptions periodUnits: periodUnits
      mask TypeOptions timerSource: timerSource
      mask TypeOptions timerPeriod_clk: timerPeriod_clk
      mask TypeOptions timerPeriod_sec: timerPeriod_sec
      mask TypeOptions tbshadow: tbshadow
      mask TypeOptions countingMode: countingMode
      mask TypeOptions phaseActiveEnable: phaseActiveEnable
      mask TypeOptions phaseDirection: phaseDirection
      mask TypeOptions phaseActive: phaseActive
      mask TypeOptions synchronizationEnable: synchronizationEnable
      mask TypeOptions dcaevt1Sync: dcaevt1Sync
      mask TypeOptions dcbevt1Sync: dcbevt1Sync
      mask TypeOptions synchronizationOption: synchronizationOption
      mask TypeOptions perSynchronizationOption: perSynchronizationOption
      mask TypeOptions clockPrescale: clockPrescale
      mask TypeOptions HSclockPrescale: HSclockPrescale
      mask TypeOptions enswap: enswap
      mask TypeOptions ePWMxAStatus: ePWMxAStatus
      mask TypeOptions ePWMxAactionLogic1: ePWMxAactionLogic1
      mask TypeOptions ePWMxAactionLogic2: ePWMxAactionLogic2
      mask TypeOptions ePWMxAactionLogic3: ePWMxAactionLogic3
      mask TypeOptions ePWMxAactionLogic4: ePWMxAactionLogic4
      mask TypeOptions ePWMxAactionLogic5: ePWMxAactionLogic5
      mask TypeOptions ePWMxAactionLogic6: ePWMxAactionLogic6
      mask TypeOptions ePWMxACSFenable: ePWMxACSFenable
      mask TypeOptions ePWMxACSFvalue: ePWMxACSFvalue
      mask TypeOptions ePWMxASFreload: ePWMxASFreload
      mask TypeOptions ePWMxBStatus: ePWMxBStatus
      mask TypeOptions ePWMxBactionLogic1: ePWMxBactionLogic1
      mask TypeOptions ePWMxBactionLogic2: ePWMxBactionLogic2
      mask TypeOptions ePWMxBactionLogic3: ePWMxBactionLogic3
      mask TypeOptions ePWMxBactionLogic4: ePWMxBactionLogic4
      mask TypeOptions ePWMxBactionLogic5: ePWMxBactionLogic5
      mask TypeOptions ePWMxBactionLogic6: ePWMxBactionLogic6
      mask TypeOptions ePWMxBCSFenable: ePWMxBCSFenable
      mask TypeOptions ePWMxBCSFvalue: ePWMxBCSFvalue
      mask TypeOptions ePWMxBSFreload: ePWMxBSFreload
      mask TypeOptions ePWNxBOutWay: ePWNxBOutWay
      mask TypeOptions ePWMxLINKCMPA: ePWMxLINKCMPA
      mask TypeOptions CMPAUnits: CMPAUnits
      mask TypeOptions CMPASource: CMPASource
      mask TypeOptions CMPAValue_per: CMPAValue_per
      mask TypeOptions CMPAValue_clk: CMPAValue_clk
      mask TypeOptions enCMPAshadow: enCMPAshadow
      mask TypeOptions ePWMxLINKCMPB: ePWMxLINKCMPB
      mask TypeOptions CMPBUnits: CMPBUnits
      mask TypeOptions CMPBSource: CMPBSource
      mask TypeOptions CMPBValue_per: CMPBValue_per
      mask TypeOptions CMPBValue_clk: CMPBValue_clk
      mask TypeOptions enCMPBshadow: enCMPBshadow
      mask TypeOptions ePWMxLINKCMPC: ePWMxLINKCMPC
      mask TypeOptions CMPCUnits: CMPCUnits
      mask TypeOptions CMPCSource: CMPCSource
      mask TypeOptions CMPCValue_per: CMPCValue_per
      mask TypeOptions CMPCValue_clk: CMPCValue_clk
      mask TypeOptions enCMPCshadow: enCMPCshadow
      mask TypeOptions ePWMxLINKCMPD: ePWMxLINKCMPD
      mask TypeOptions CMPDUnits: CMPDUnits
      mask TypeOptions CMPDSource: CMPDSource
      mask TypeOptions CMPDValue_per: CMPDValue_per
      mask TypeOptions CMPDValue_clk: CMPDValue_clk
      mask TypeOptions enCMPDshadow: enCMPDshadow
      mask TypeOptions enableDBePWMxA: enableDBePWMxA
      mask TypeOptions enableDBePWMxB: enableDBePWMxB
      mask TypeOptions enhalfcycle: enhalfcycle
      mask TypeOptions DBpolarity: DBpolarity
      mask TypeOptions DBedgeDelay: DBedgeDelay
      mask TypeOptions DBSource_ePWMxA: DBSource_ePWMxA
      mask TypeOptions DBSource_ePWMxB: DBSource_ePWMxB
      mask TypeOptions DBPeriodUnits: DBPeriodUnits
      mask TypeOptions DBperiodSource: DBperiodSource
      mask TypeOptions REDperiod: REDperiod
      mask TypeOptions FEDperiod: FEDperiod
      mask TypeOptions REDperiod_sec: REDperiod_sec
      mask TypeOptions FEDperiod_sec: FEDperiod_sec
      mask TypeOptions LoadModeDBRED: LoadModeDBRED
      mask TypeOptions LoadModeDBFED: LoadModeDBFED
      mask TypeOptions adcstartModuleA: adcstartModuleA
      mask TypeOptions adcrequestEventA: adcrequestEventA
      mask TypeOptions adcstartEventA: adcstartEventA
      mask TypeOptions adcstartEventA_type2: adcstartEventA_type2
      mask TypeOptions adcstartModuleB: adcstartModuleB
      mask TypeOptions adcrequestEventB: adcrequestEventB
      mask TypeOptions adcstartEventB: adcstartEventB
      mask TypeOptions adcstartEventB_type2: adcstartEventB_type2
      mask TypeOptions intEn: intEn
      mask TypeOptions intPrd: intPrd
      mask TypeOptions intSel: intSel
      mask TypeOptions intSel_type2: intSel_type2
      mask TypeOptions hrpe: hrpe
      mask TypeOptions enHRPWM: enHRPWM
      mask TypeOptions HRPWM_LoadMode: HRPWM_LoadMode
      mask TypeOptions HRPWM_CTLMode: HRPWM_CTLMode
      mask TypeOptions HRPWM_EDGMode: HRPWM_EDGMode
      mask TypeOptions hrpeb: hrpeb
      mask TypeOptions enHRPWMB: enHRPWMB
      mask TypeOptions HRPWM_LoadModeB: HRPWM_LoadModeB
      mask TypeOptions HRPWM_CTLModeB: HRPWM_CTLModeB
      mask TypeOptions HRPWM_EDGModeB: HRPWM_EDGModeB
      mask TypeOptions enHRDBRED: enHRDBRED
      mask TypeOptions enHRDBFED: enHRDBFED
      mask TypeOptions enSFO: enSFO
      mask TypeOptions enautoconv: enautoconv
      mask TypeOptions chopperEnable: chopperEnable
      mask TypeOptions chopperFrequency: chopperFrequency
      mask TypeOptions chopperFirstwidth: chopperFirstwidth
      mask TypeOptions chopperDuty: chopperDuty
      mask TypeOptions tripZonesource: tripZonesource
      mask TypeOptions tzselOSHT1: tzselOSHT1
      mask TypeOptions tzselOSHT2: tzselOSHT2
      mask TypeOptions tzselOSHT3: tzselOSHT3
      mask TypeOptions tzselOSHDCAEV1: tzselOSHDCAEV1
      mask TypeOptions tzselOSHDCBEV1: tzselOSHDCBEV1
      mask TypeOptions tzselCBC1: tzselCBC1
      mask TypeOptions tzselCBC2: tzselCBC2
      mask TypeOptions tzselCBC3: tzselCBC3
      mask TypeOptions tzselCBCDCAEV2: tzselCBCDCAEV2
      mask TypeOptions tzselCBCDCBEV2: tzselCBCDCBEV2
      mask TypeOptions tzselOSHT4: tzselOSHT4
      mask TypeOptions tzselOSHT5: tzselOSHT5
      mask TypeOptions tzselOSHT6: tzselOSHT6
      mask TypeOptions tzselCBC4: tzselCBC4
      mask TypeOptions tzselCBC5: tzselCBC5
      mask TypeOptions tzselCBC6: tzselCBC6
      mask TypeOptions enTzOstIntr: enTzOstIntr
      mask TypeOptions enTzCbcIntr: enTzCbcIntr
      mask TypeOptions enTzDCAEVT1Intr: enTzDCAEVT1Intr
      mask TypeOptions enTzDCAEVT2Intr: enTzDCAEVT2Intr
      mask TypeOptions enTzDCBEVT1Intr: enTzDCBEVT1Intr
      mask TypeOptions enTzDCBEVT2Intr: enTzDCBEVT2Intr
      mask TypeOptions ePWMxAforced: ePWMxAforced
      mask TypeOptions ePWMxBforced: ePWMxBforced
      mask TypeOptions DCAEVT1forced: DCAEVT1forced
      mask TypeOptions DCBEVT1forced: DCBEVT1forced
      mask TypeOptions DCAEVT2forced: DCAEVT2forced
      mask TypeOptions DCBEVT2forced: DCBEVT2forced
      mask TypeOptions dcah: dcah
      mask TypeOptions dcal: dcal
      mask TypeOptions dcbh: dcbh
      mask TypeOptions dcbl: dcbl
      mask TypeOptions dcah_type2: dcah_type2
      mask TypeOptions dcal_type2: dcal_type2
      mask TypeOptions dcbh_type2: dcbh_type2
      mask TypeOptions dcbl_type2: dcbl_type2
      mask TypeOptions gendcaevt1: gendcaevt1
      mask TypeOptions gendcaevt2: gendcaevt2
      mask TypeOptions gendcbevt1: gendcbevt1
      mask TypeOptions gendcbevt2: gendcbevt2
      mask TypeOptions dcaevt1src: dcaevt1src
      mask TypeOptions dcaevt2src: dcaevt2src
      mask TypeOptions dcbevt1src: dcbevt1src
      mask TypeOptions dcbevt2src: dcbevt2src
      mask TypeOptions pulsesel: pulsesel
      mask TypeOptions blankinv: blankinv
      mask TypeOptions blankoffset: blankoffset
      mask TypeOptions blankwidth: blankwidth
      mask TypeOptions evsrcsel: evsrcsel
      mask TypeOptions encape: encape
  wires:
  MOSFET_Timer/1 -> ePWM2_MOSFET/1
  Demux/2 -> Rate Transition8/1
  Rate Transition9/1 -> BlueLED/1
  Demux/1 -> Rate Transition10/1
  Rate Transition3/1 -> ePWM2_MOSFET/3
  Demux/3 -> Rate Transition9/1
  Rate Transition7/1 -> ePWM1_IGBT/3
  Rate Transition8/1 -> GreenLED/1
  Rate Transition10/1 -> RedLED/1
  MOSFET_DUTY_CYCLE/1 -> ePWM2_MOSFET/2
  IGBT_Timer/1 -> ePWM1_IGBT/1
  IGBT_ENABLE/1 -> Rate Transition7/1
  IGBT_DUTY_CYCLE/1 -> ePWM1_IGBT/2
  MOSFET_ENABLE/1 -> Rate Transition3/1
  LED/1 -> Demux/1

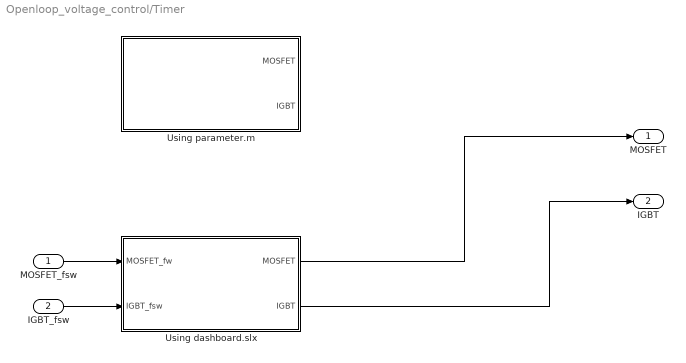
== system Openloop_voltage_control/Timer ==
  MOSFET_fsw : Inport
  IGBT_fsw : Inport  Port=2
  Using dashboard.slx : Subsystem
  Using parameter.m : Subsystem
  MOSFET : Outport
  IGBT : Outport  Port=2
  wires:
  MOSFET_fsw/1 -> Using dashboard.slx/1(MOSFET_fw)
  IGBT_fsw/1 -> Using dashboard.slx/2(IGBT_fsw)
  Using dashboard.slx/1(MOSFET) -> MOSFET/1
  Using dashboard.slx/2(IGBT) -> IGBT/1
